simulink model "test_matlab_system_19"  (Simulink 10.2)
settings: Solver=FixedStepAuto  StartTime=0.0  StopTime=Config.simulationTime  FixedStep=Config.tStep  RelTol=1e-3
PostLoadFcn:
  | % Set path to the utility functions and to WBC library
  | import wbc.*
  | addpath(genpath('./src'));
  | addpath('./lib/RobotDynamicsWithContacts');
InitFcn:
  | init
undefined symbols (not defined in the file or in its folder): Config, confVisualizer, robot_config
libraries: WBToolboxLibrary x1, robotDynamicsWithContacts_lib x1
settings Model: Creator=giuseppe  LastModifiedBy=nunoguedelha
settings DataIOCC: SaveFormat=Dataset  SignalLoggingSaveFormat=Dataset  ReturnWorkspaceOutputs=on
settings OptimizationCC: LifeSpan=auto
settings DebuggingCC: UnderspecifiedInitializationDetection=Simplified  MergeDetectMultiDrivingBlocksExec=error  FcnCallInpInsideContextMsg=error  SFUnexpectedBacktrackingDiag=error  SFNoUnconditionalDefaultTransitionDiag=error  SFExecutionAtInitializationDiag=warning  ArithmeticOperatorsInVariantConditions=error
settings HardwareCC: ProdBitPerPointer=64  ProdBitPerSizeT=64  ProdBitPerPtrDiffT=64  ProdLargestAtomicFloat=Float  ProdIntDivRoundTo=Zero  ProdEndianess=LittleEndian  ProdWordSize=64  ProdHWDeviceType=Intel->x86-64 (Windows64)
settings ModelReferenceCC: PropagateSignalLabelsOutOfModel=on
settings SFSimCC: SimUseLocalCustomCode=on  CustomCodeUndefinedFunction=FilterOut
settings RTWCC: RTWUseLocalCustomCode=on
settings CodeAppCC: StateflowObjectComments=off
settings GRTTargetCC: TargetLangStandard=C99 (ISO)  CombineOutputUpdateFcns=on  GRTInterface=off
settings ConfigComp: CovMetricSettings=dwe  CovSaveCumulativeToWorkspaceVar=off  CovSaveSingleToWorkspaceVar=off  CovExternalEMLEnable=on

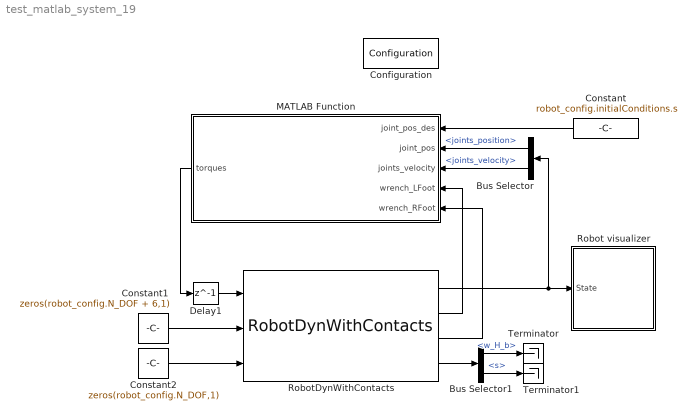
== system test_matlab_system_19 ==
  Bus Selector : BusSelector  OutputSignals=joints_position,joints_velocity
  Bus Selector1 : BusSelector  OutputSignals=w_H_b,s
  Configuration : WBToolboxLibrary/Utilities/Configuration  ConfigSource=Workspace  ConfigObject='WBTConfigRobotSim'  RobotName='icubSim'  UrdfFile='model.urdf'  ControlledJoints={'l_elbow','l_shoulder_pitch','torso_roll'}  ControlBoardsNames={'left_arm','right_arm','torso'}  LocalName='WBT'  GravityVector=[0,0,-9.81]
      settings: SourceProductName=WholeBodyToolbox
  Constant : Constant  Value=robot_config.initialConditions.s
  Constant1 : Constant  Value=zeros(robot_config.N_DOF + 6,1)
  Constant2 : Constant  Value=zeros(robot_config.N_DOF,1)
  Delay1 : Delay  DelayLength=1  InitialCondition=zeros(23,1)
  MATLAB Function : MATLAB Function  TreatAsAtomicUnit=on  SystemSampleTime=Config.tStep
  Robot visualizer : Subsystem  TreatAsAtomicUnit=on  SystemSampleTime=confVisualizer.tStep
  RobotDynWithContacts : robotDynamicsWithContacts_lib/RobotDynWithContacts  robot_config=robot_config  contact_config=contact_config  physics_config=physics_config
      settings: SourceProductName=RobotDynamicsWithContacts
  Terminator : Terminator
  Terminator1 : Terminator
  wires:
  Constant1/1 -> RobotDynWithContacts/2
  Bus Selector/1 -> MATLAB Function/2(joint_pos)  "<joints_position>"
  Bus Selector/2 -> MATLAB Function/3(joints_velocity)  "<joints_velocity>"
  RobotDynWithContacts/1 -> Robot visualizer/1(State), Bus Selector/1
  RobotDynWithContacts/2 -> MATLAB Function/4(wrench_LFoot)
  RobotDynWithContacts/3 -> MATLAB Function/5(wrench_RFoot)
  Constant/1 -> MATLAB Function/1(joint_pos_des)
  MATLAB Function/1(torques) -> Delay1/1
  Delay1/1 -> RobotDynWithContacts/1
  RobotDynWithContacts/4 -> Bus Selector1/1
  Bus Selector1/2 -> Terminator1/1  "<s>"
  Bus Selector1/1 -> Terminator/1  "<w_H_b>"
  Constant2/1 -> RobotDynWithContacts/3

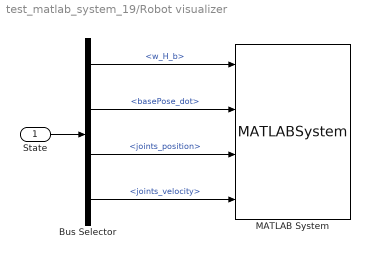
== system test_matlab_system_19/Robot visualizer ==
  State : Inport
  Bus Selector : BusSelector  OutputSignals=w_H_b,basePose_dot,joints_position,joints_velocity
  MATLAB System : MATLABSystem  System=Visualizer  config=confVisualizer  SimulateUsing=Interpreted execution
      mask Type: Visualizer
      mask Display:
      | disp(['Robot' char(10) 'Visualizer']);
      | port_label('input',1,'world_H_base');
      | port_label('input',2,'base_velocity');
      | port_label('input',3,'joints_positions');
      | port_label('input',4,'joints_velocity');
  wires:
  State/1 -> Bus Selector/1
  Bus Selector/1 -> MATLAB System/1  "<w_H_b>"
  Bus Selector/3 -> MATLAB System/3  "<joints_position>"
  Bus Selector/2 -> MATLAB System/2  "<basePose_dot>"
  Bus Selector/4 -> MATLAB System/4  "<joints_velocity>"

== matlab function MATLAB Function ==
  data: torques output double; joint_pos_des input double; joint_pos input double; joints_velocity input double; wrench_LFoot input double; wrench_RFoot input double
function torques = dummy_torque_control(joint_pos_des, joint_pos, joints_velocity, wrench_LFoot, wrench_RFoot)
    
    joints_pos_error = (joint_pos_des - joint_pos);
    
    KP = 0.1;
    KD = 2*sqrt(KP);
    
    torques = KP*(joints_pos_error) - KD*joints_velocity;
